simulink model "l512_devel_pps_2016f"  (R2012b)
settings: Solver=ode45  StartTime=0.0  StopTime=15000  RelTol=1e-3
undefined symbols (not defined in the file): sfp
libraries: xbsIndex_r4 x7383, casper_library_misc x259, casper_library_delays x118, xps_library x12, simulink x1
(part 5 of 82)

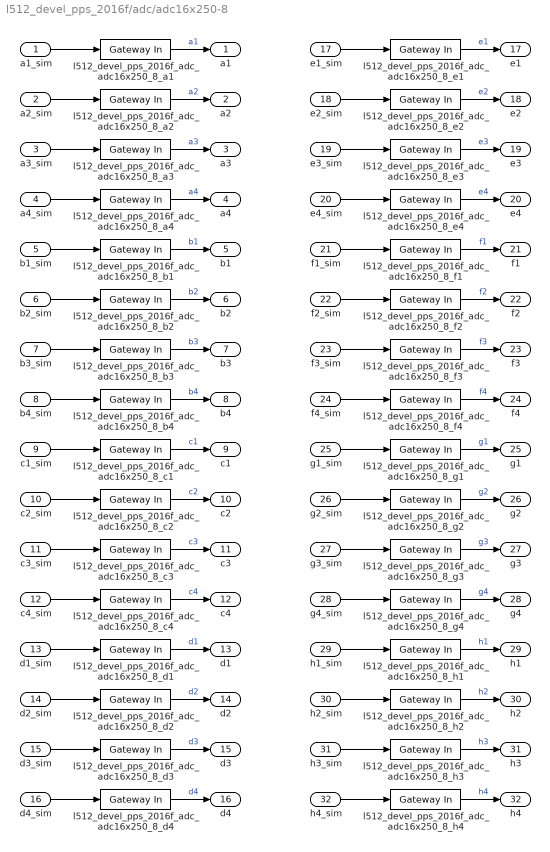
== system l512_devel_pps_2016f/adc/adc16x250-8 ==
  a1_sim : Inport
  a2_sim : Inport  Port=2
  a3_sim : Inport  Port=3
  a4_sim : Inport  Port=4
  b1_sim : Inport  Port=5
  b2_sim : Inport  Port=6
  b3_sim : Inport  Port=7
  b4_sim : Inport  Port=8
  c1_sim : Inport  Port=9
  c2_sim : Inport  Port=10
  c3_sim : Inport  Port=11
  c4_sim : Inport  Port=12
  d1_sim : Inport  Port=13
  d2_sim : Inport  Port=14
  d3_sim : Inport  Port=15
  d4_sim : Inport  Port=16
  e1_sim : Inport  Port=17
  e2_sim : Inport  Port=18
  e3_sim : Inport  Port=19
  e4_sim : Inport  Port=20
  f1_sim : Inport  Port=21
  f2_sim : Inport  Port=22
  f3_sim : Inport  Port=23
  f4_sim : Inport  Port=24
  g1_sim : Inport  Port=25
  g2_sim : Inport  Port=26
  g3_sim : Inport  Port=27
  g4_sim : Inport  Port=28
  h1_sim : Inport  Port=29
  h2_sim : Inport  Port=30
  h3_sim : Inport  Port=31
  h4_sim : Inport  Port=32
  l512_devel_pps_2016f_adc_adc16x250_8_a{1..4} (4 alike) : xbsIndex_r4/Gateway In  gui_display_data_type=Fixed-point  arith_type="Signed  (2's comp)"  n_bits=8  bin_pt=7  preci_type=Single  exp_width=8  frac_width=24  quantization="Round  (unbiased: +/- Inf)"  overflow=Saturate  period=1  dbl_ovrd=off  timing_constraint=None  locs_specified=off  LOCs={}  UseAsADC=off  ADCChannel='1'  inherit_from_input=off  hdl_port=on  block_type=gatewayin
  l512_devel_pps_2016f_adc_adc16x250_8_b{1..4} (4 alike) : xbsIndex_r4/Gateway In  gui_display_data_type=Fixed-point  arith_type="Signed  (2's comp)"  n_bits=8  bin_pt=7  preci_type=Single  exp_width=8  frac_width=24  quantization="Round  (unbiased: +/- Inf)"  overflow=Saturate  period=1  dbl_ovrd=off  timing_constraint=None  locs_specified=off  LOCs={}  UseAsADC=off  ADCChannel='1'  inherit_from_input=off  hdl_port=on  block_type=gatewayin
  l512_devel_pps_2016f_adc_adc16x250_8_c{1..4} (4 alike) : xbsIndex_r4/Gateway In  gui_display_data_type=Fixed-point  arith_type="Signed  (2's comp)"  n_bits=8  bin_pt=7  preci_type=Single  exp_width=8  frac_width=24  quantization="Round  (unbiased: +/- Inf)"  overflow=Saturate  period=1  dbl_ovrd=off  timing_constraint=None  locs_specified=off  LOCs={}  UseAsADC=off  ADCChannel='1'  inherit_from_input=off  hdl_port=on  block_type=gatewayin
  l512_devel_pps_2016f_adc_adc16x250_8_d{1..4} (4 alike) : xbsIndex_r4/Gateway In  gui_display_data_type=Fixed-point  arith_type="Signed  (2's comp)"  n_bits=8  bin_pt=7  preci_type=Single  exp_width=8  frac_width=24  quantization="Round  (unbiased: +/- Inf)"  overflow=Saturate  period=1  dbl_ovrd=off  timing_constraint=None  locs_specified=off  LOCs={}  UseAsADC=off  ADCChannel='1'  inherit_from_input=off  hdl_port=on  block_type=gatewayin
  l512_devel_pps_2016f_adc_adc16x250_8_e{1..4} (4 alike) : xbsIndex_r4/Gateway In  gui_display_data_type=Fixed-point  arith_type="Signed  (2's comp)"  n_bits=8  bin_pt=7  preci_type=Single  exp_width=8  frac_width=24  quantization="Round  (unbiased: +/- Inf)"  overflow=Saturate  period=1  dbl_ovrd=off  timing_constraint=None  locs_specified=off  LOCs={}  UseAsADC=off  ADCChannel='1'  inherit_from_input=off  hdl_port=on  block_type=gatewayin
  l512_devel_pps_2016f_adc_adc16x250_8_f{1..4} (4 alike) : xbsIndex_r4/Gateway In  gui_display_data_type=Fixed-point  arith_type="Signed  (2's comp)"  n_bits=8  bin_pt=7  preci_type=Single  exp_width=8  frac_width=24  quantization="Round  (unbiased: +/- Inf)"  overflow=Saturate  period=1  dbl_ovrd=off  timing_constraint=None  locs_specified=off  LOCs={}  UseAsADC=off  ADCChannel='1'  inherit_from_input=off  hdl_port=on  block_type=gatewayin
  l512_devel_pps_2016f_adc_adc16x250_8_g{1..4} (4 alike) : xbsIndex_r4/Gateway In  gui_display_data_type=Fixed-point  arith_type="Signed  (2's comp)"  n_bits=8  bin_pt=7  preci_type=Single  exp_width=8  frac_width=24  quantization="Round  (unbiased: +/- Inf)"  overflow=Saturate  period=1  dbl_ovrd=off  timing_constraint=None  locs_specified=off  LOCs={}  UseAsADC=off  ADCChannel='1'  inherit_from_input=off  hdl_port=on  block_type=gatewayin
  l512_devel_pps_2016f_adc_adc16x250_8_h{1..4} (4 alike) : xbsIndex_r4/Gateway In  gui_display_data_type=Fixed-point  arith_type="Signed  (2's comp)"  n_bits=8  bin_pt=7  preci_type=Single  exp_width=8  frac_width=24  quantization="Round  (unbiased: +/- Inf)"  overflow=Saturate  period=1  dbl_ovrd=off  timing_constraint=None  locs_specified=off  LOCs={}  UseAsADC=off  ADCChannel='1'  inherit_from_input=off  hdl_port=on  block_type=gatewayin
  a1 : Outport
  a2 : Outport  Port=2
  a3 : Outport  Port=3
  a4 : Outport  Port=4
  b1 : Outport  Port=5
  b2 : Outport  Port=6
  b3 : Outport  Port=7
  b4 : Outport  Port=8
  c1 : Outport  Port=9
  c2 : Outport  Port=10
  c3 : Outport  Port=11
  c4 : Outport  Port=12
  d1 : Outport  Port=13
  d2 : Outport  Port=14
  d3 : Outport  Port=15
  d4 : Outport  Port=16
  e1 : Outport  Port=17
  e2 : Outport  Port=18
  e3 : Outport  Port=19
  e4 : Outport  Port=20
  f1 : Outport  Port=21
  f2 : Outport  Port=22
  f3 : Outport  Port=23
  f4 : Outport  Port=24
  g1 : Outport  Port=25
  g2 : Outport  Port=26
  g3 : Outport  Port=27
  g4 : Outport  Port=28
  h1 : Outport  Port=29
  h2 : Outport  Port=30
  h3 : Outport  Port=31
  h4 : Outport  Port=32
  wires:
  a1_sim/1 -> l512_devel_pps_2016f_adc_adc16x250_8_a1/1
  l512_devel_pps_2016f_adc_adc16x250_8_a1/1 -> a1/1  "a1"
  a2_sim/1 -> l512_devel_pps_2016f_adc_adc16x250_8_a2/1
  l512_devel_pps_2016f_adc_adc16x250_8_a2/1 -> a2/1  "a2"
  a3_sim/1 -> l512_devel_pps_2016f_adc_adc16x250_8_a3/1
  l512_devel_pps_2016f_adc_adc16x250_8_a3/1 -> a3/1  "a3"
  a4_sim/1 -> l512_devel_pps_2016f_adc_adc16x250_8_a4/1
  l512_devel_pps_2016f_adc_adc16x250_8_a4/1 -> a4/1  "a4"
  b1_sim/1 -> l512_devel_pps_2016f_adc_adc16x250_8_b1/1
  l512_devel_pps_2016f_adc_adc16x250_8_b1/1 -> b1/1  "b1"
  b2_sim/1 -> l512_devel_pps_2016f_adc_adc16x250_8_b2/1
  l512_devel_pps_2016f_adc_adc16x250_8_b2/1 -> b2/1  "b2"
  b3_sim/1 -> l512_devel_pps_2016f_adc_adc16x250_8_b3/1
  l512_devel_pps_2016f_adc_adc16x250_8_b3/1 -> b3/1  "b3"
  b4_sim/1 -> l512_devel_pps_2016f_adc_adc16x250_8_b4/1
  l512_devel_pps_2016f_adc_adc16x250_8_b4/1 -> b4/1  "b4"
  c1_sim/1 -> l512_devel_pps_2016f_adc_adc16x250_8_c1/1
  l512_devel_pps_2016f_adc_adc16x250_8_c1/1 -> c1/1  "c1"
  c2_sim/1 -> l512_devel_pps_2016f_adc_adc16x250_8_c2/1
  l512_devel_pps_2016f_adc_adc16x250_8_c2/1 -> c2/1  "c2"
  c3_sim/1 -> l512_devel_pps_2016f_adc_adc16x250_8_c3/1
  l512_devel_pps_2016f_adc_adc16x250_8_c3/1 -> c3/1  "c3"
  c4_sim/1 -> l512_devel_pps_2016f_adc_adc16x250_8_c4/1
  l512_devel_pps_2016f_adc_adc16x250_8_c4/1 -> c4/1  "c4"
  d1_sim/1 -> l512_devel_pps_2016f_adc_adc16x250_8_d1/1
  l512_devel_pps_2016f_adc_adc16x250_8_d1/1 -> d1/1  "d1"
  d2_sim/1 -> l512_devel_pps_2016f_adc_adc16x250_8_d2/1
  l512_devel_pps_2016f_adc_adc16x250_8_d2/1 -> d2/1  "d2"
  d3_sim/1 -> l512_devel_pps_2016f_adc_adc16x250_8_d3/1
  l512_devel_pps_2016f_adc_adc16x250_8_d3/1 -> d3/1  "d3"
  d4_sim/1 -> l512_devel_pps_2016f_adc_adc16x250_8_d4/1
  l512_devel_pps_2016f_adc_adc16x250_8_d4/1 -> d4/1  "d4"
  e1_sim/1 -> l512_devel_pps_2016f_adc_adc16x250_8_e1/1
  l512_devel_pps_2016f_adc_adc16x250_8_e1/1 -> e1/1  "e1"
  e2_sim/1 -> l512_devel_pps_2016f_adc_adc16x250_8_e2/1
  l512_devel_pps_2016f_adc_adc16x250_8_e2/1 -> e2/1  "e2"
  e3_sim/1 -> l512_devel_pps_2016f_adc_adc16x250_8_e3/1
  l512_devel_pps_2016f_adc_adc16x250_8_e3/1 -> e3/1  "e3"
  e4_sim/1 -> l512_devel_pps_2016f_adc_adc16x250_8_e4/1
  l512_devel_pps_2016f_adc_adc16x250_8_e4/1 -> e4/1  "e4"
  f1_sim/1 -> l512_devel_pps_2016f_adc_adc16x250_8_f1/1
  l512_devel_pps_2016f_adc_adc16x250_8_f1/1 -> f1/1  "f1"
  f2_sim/1 -> l512_devel_pps_2016f_adc_adc16x250_8_f2/1
  l512_devel_pps_2016f_adc_adc16x250_8_f2/1 -> f2/1  "f2"
  f3_sim/1 -> l512_devel_pps_2016f_adc_adc16x250_8_f3/1
  l512_devel_pps_2016f_adc_adc16x250_8_f3/1 -> f3/1  "f3"
  f4_sim/1 -> l512_devel_pps_2016f_adc_adc16x250_8_f4/1
  l512_devel_pps_2016f_adc_adc16x250_8_f4/1 -> f4/1  "f4"
  g1_sim/1 -> l512_devel_pps_2016f_adc_adc16x250_8_g1/1
  l512_devel_pps_2016f_adc_adc16x250_8_g1/1 -> g1/1  "g1"
  g2_sim/1 -> l512_devel_pps_2016f_adc_adc16x250_8_g2/1
  l512_devel_pps_2016f_adc_adc16x250_8_g2/1 -> g2/1  "g2"
  g3_sim/1 -> l512_devel_pps_2016f_adc_adc16x250_8_g3/1
  l512_devel_pps_2016f_adc_adc16x250_8_g3/1 -> g3/1  "g3"
  g4_sim/1 -> l512_devel_pps_2016f_adc_adc16x250_8_g4/1
  l512_devel_pps_2016f_adc_adc16x250_8_g4/1 -> g4/1  "g4"
  h1_sim/1 -> l512_devel_pps_2016f_adc_adc16x250_8_h1/1
  l512_devel_pps_2016f_adc_adc16x250_8_h1/1 -> h1/1  "h1"
  h2_sim/1 -> l512_devel_pps_2016f_adc_adc16x250_8_h2/1
  l512_devel_pps_2016f_adc_adc16x250_8_h2/1 -> h2/1  "h2"
  h3_sim/1 -> l512_devel_pps_2016f_adc_adc16x250_8_h3/1
  l512_devel_pps_2016f_adc_adc16x250_8_h3/1 -> h3/1  "h3"
  h4_sim/1 -> l512_devel_pps_2016f_adc_adc16x250_8_h4/1
  l512_devel_pps_2016f_adc_adc16x250_8_h4/1 -> h4/1  "h4"

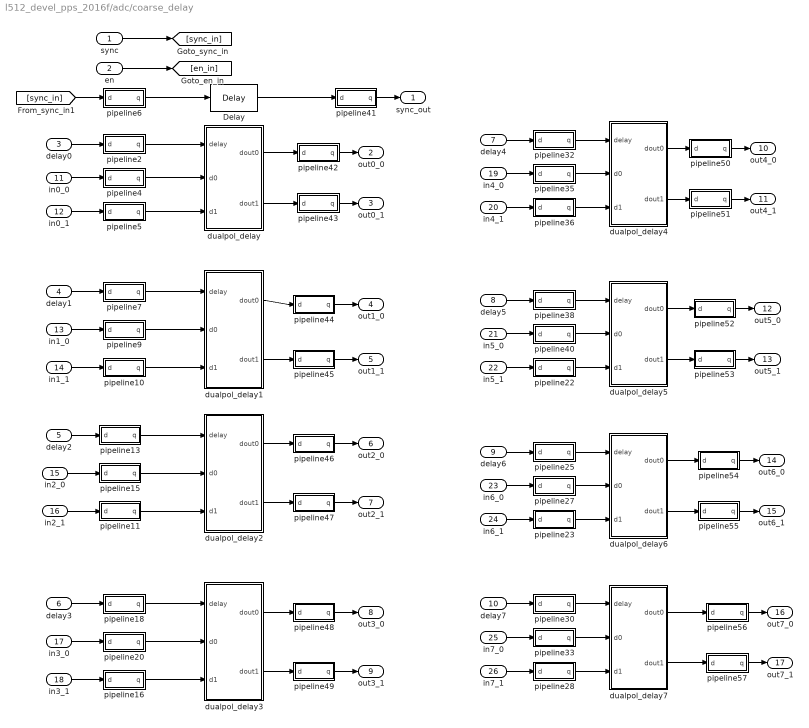
== system l512_devel_pps_2016f/adc/coarse_delay ==
  sync : Inport
  en : Inport  Port=2
  delay0 : Inport  Port=3
  delay1 : Inport  Port=4
  delay2 : Inport  Port=5
  delay3 : Inport  Port=6
  delay4 : Inport  Port=7
  delay5 : Inport  Port=8
  delay6 : Inport  Port=9
  delay7 : Inport  Port=10
  in0_0 : Inport  Port=11
  in0_1 : Inport  Port=12
  in1_0 : Inport  Port=13
  in1_1 : Inport  Port=14
  in2_0 : Inport  Port=15
  in2_1 : Inport  Port=16
  in3_0 : Inport  Port=17
  in3_1 : Inport  Port=18
  in4_0 : Inport  Port=19
  in4_1 : Inport  Port=20
  in5_0 : Inport  Port=21
  in5_1 : Inport  Port=22
  in6_0 : Inport  Port=23
  in6_1 : Inport  Port=24
  in7_0 : Inport  Port=25
  in7_1 : Inport  Port=26
  Delay : xbsIndex_r4/Delay  rst=off  infoeditControl=Selection of Reset will increase slice count due to use of real FFs and instead of SRLs  en=off  latency=3  dbl_ovrd=off  reg_retiming=off  block_type=delay
  dualpol_delay : Subsystem
  dualpol_delay1 : Subsystem
  dualpol_delay2 : Subsystem
  dualpol_delay3 : Subsystem
  dualpol_delay4 : Subsystem
  dualpol_delay5 : Subsystem
  dualpol_delay6 : Subsystem
  dualpol_delay7 : Subsystem
  pipeline10 : Subsystem  AncestorBlock=casper_library_delays/pipeline  mask(pipeline){latency=1}
      mask help:
      | An explicitly laid-out delay line to avoid mapping to SRL16s
      | for use in pipelining to help achieve timing closure.
      mask init:
      | pipeline_init(gcb,'latency',latency);
      settings: AttributesFormatString=Latency = %<latency>
      mask Display:
      | port_label('input', 1, 'd');
      | port_label('output', 1, 'q');
      | disp(['Z^-', num2str(latency)]);
  pipeline11 : Subsystem  AncestorBlock=casper_library_delays/pipeline  mask(pipeline){latency=1}
      mask help:
      | An explicitly laid-out delay line to avoid mapping to SRL16s
      | for use in pipelining to help achieve timing closure.
      mask init:
      | pipeline_init(gcb,'latency',latency);
      settings: AttributesFormatString=Latency = %<latency>
      mask Display:
      | port_label('input', 1, 'd');
      | port_label('output', 1, 'q');
      | disp(['Z^-', num2str(latency)]);
  pipeline13 : Subsystem  AncestorBlock=casper_library_delays/pipeline  mask(pipeline){latency=1}
      mask help:
      | An explicitly laid-out delay line to avoid mapping to SRL16s
      | for use in pipelining to help achieve timing closure.
      mask init:
      | pipeline_init(gcb,'latency',latency);
      settings: AttributesFormatString=Latency = %<latency>
      mask Display:
      | port_label('input', 1, 'd');
      | port_label('output', 1, 'q');
      | disp(['Z^-', num2str(latency)]);
  pipeline15 : Subsystem  AncestorBlock=casper_library_delays/pipeline  mask(pipeline){latency=1}
      mask help:
      | An explicitly laid-out delay line to avoid mapping to SRL16s
      | for use in pipelining to help achieve timing closure.
      mask init:
      | pipeline_init(gcb,'latency',latency);
      settings: AttributesFormatString=Latency = %<latency>
      mask Display:
      | port_label('input', 1, 'd');
      | port_label('output', 1, 'q');
      | disp(['Z^-', num2str(latency)]);
  pipeline16 : Subsystem  AncestorBlock=casper_library_delays/pipeline  mask(pipeline){latency=1}
      mask help:
      | An explicitly laid-out delay line to avoid mapping to SRL16s
      | for use in pipelining to help achieve timing closure.
      mask init:
      | pipeline_init(gcb,'latency',latency);
      settings: AttributesFormatString=Latency = %<latency>
      mask Display:
      | port_label('input', 1, 'd');
      | port_label('output', 1, 'q');
      | disp(['Z^-', num2str(latency)]);
  pipeline18 : Subsystem  AncestorBlock=casper_library_delays/pipeline  mask(pipeline){latency=1}
      mask help:
      | An explicitly laid-out delay line to avoid mapping to SRL16s
      | for use in pipelining to help achieve timing closure.
      mask init:
      | pipeline_init(gcb,'latency',latency);
      settings: AttributesFormatString=Latency = %<latency>
      mask Display:
      | port_label('input', 1, 'd');
      | port_label('output', 1, 'q');
      | disp(['Z^-', num2str(latency)]);
  pipeline2 : Subsystem  AncestorBlock=casper_library_delays/pipeline  mask(pipeline){latency=1}
      mask help:
      | An explicitly laid-out delay line to avoid mapping to SRL16s
      | for use in pipelining to help achieve timing closure.
      mask init:
      | pipeline_init(gcb,'latency',latency);
      settings: AttributesFormatString=Latency = %<latency>
      mask Display:
      | port_label('input', 1, 'd');
      | port_label('output', 1, 'q');
      | disp(['Z^-', num2str(latency)]);
  pipeline20 : Subsystem  AncestorBlock=casper_library_delays/pipeline  mask(pipeline){latency=1}
      mask help:
      | An explicitly laid-out delay line to avoid mapping to SRL16s
      | for use in pipelining to help achieve timing closure.
      mask init:
      | pipeline_init(gcb,'latency',latency);
      settings: AttributesFormatString=Latency = %<latency>
      mask Display:
      | port_label('input', 1, 'd');
      | port_label('output', 1, 'q');
      | disp(['Z^-', num2str(latency)]);
  pipeline22 : Subsystem  AncestorBlock=casper_library_delays/pipeline  mask(pipeline){latency=1}
      mask help:
      | An explicitly laid-out delay line to avoid mapping to SRL16s
      | for use in pipelining to help achieve timing closure.
      mask init:
      | pipeline_init(gcb,'latency',latency);
      settings: AttributesFormatString=Latency = %<latency>
      mask Display:
      | port_label('input', 1, 'd');
      | port_label('output', 1, 'q');
      | disp(['Z^-', num2str(latency)]);
  pipeline23 : Subsystem  AncestorBlock=casper_library_delays/pipeline  mask(pipeline){latency=1}
      mask help:
      | An explicitly laid-out delay line to avoid mapping to SRL16s
      | for use in pipelining to help achieve timing closure.
      mask init:
      | pipeline_init(gcb,'latency',latency);
      settings: AttributesFormatString=Latency = %<latency>
      mask Display:
      | port_label('input', 1, 'd');
      | port_label('output', 1, 'q');
      | disp(['Z^-', num2str(latency)]);
  pipeline25 : Subsystem  AncestorBlock=casper_library_delays/pipeline  mask(pipeline){latency=1}
      mask help:
      | An explicitly laid-out delay line to avoid mapping to SRL16s
      | for use in pipelining to help achieve timing closure.
      mask init:
      | pipeline_init(gcb,'latency',latency);
      settings: AttributesFormatString=Latency = %<latency>
      mask Display:
      | port_label('input', 1, 'd');
      | port_label('output', 1, 'q');
      | disp(['Z^-', num2str(latency)]);
  pipeline27 : Subsystem  AncestorBlock=casper_library_delays/pipeline  mask(pipeline){latency=1}
      mask help:
      | An explicitly laid-out delay line to avoid mapping to SRL16s
      | for use in pipelining to help achieve timing closure.
      mask init:
      | pipeline_init(gcb,'latency',latency);
      settings: AttributesFormatString=Latency = %<latency>
      mask Display:
      | port_label('input', 1, 'd');
      | port_label('output', 1, 'q');
      | disp(['Z^-', num2str(latency)]);
  pipeline28 : Subsystem  AncestorBlock=casper_library_delays/pipeline  mask(pipeline){latency=1}
      mask help:
      | An explicitly laid-out delay line to avoid mapping to SRL16s
      | for use in pipelining to help achieve timing closure.
      mask init:
      | pipeline_init(gcb,'latency',latency);
      settings: AttributesFormatString=Latency = %<latency>
      mask Display:
      | port_label('input', 1, 'd');
      | port_label('output', 1, 'q');
      | disp(['Z^-', num2str(latency)]);
  pipeline30 : Subsystem  AncestorBlock=casper_library_delays/pipeline  mask(pipeline){latency=1}
      mask help:
      | An explicitly laid-out delay line to avoid mapping to SRL16s
      | for use in pipelining to help achieve timing closure.
      mask init:
      | pipeline_init(gcb,'latency',latency);
      settings: AttributesFormatString=Latency = %<latency>
      mask Display:
      | port_label('input', 1, 'd');
      | port_label('output', 1, 'q');
      | disp(['Z^-', num2str(latency)]);
  pipeline32 : Subsystem  AncestorBlock=casper_library_delays/pipeline  mask(pipeline){latency=1}
      mask help:
      | An explicitly laid-out delay line to avoid mapping to SRL16s
      | for use in pipelining to help achieve timing closure.
      mask init:
      | pipeline_init(gcb,'latency',latency);
      settings: AttributesFormatString=Latency = %<latency>
      mask Display:
      | port_label('input', 1, 'd');
      | port_label('output', 1, 'q');
      | disp(['Z^-', num2str(latency)]);
  pipeline33 : Subsystem  AncestorBlock=casper_library_delays/pipeline  mask(pipeline){latency=1}
      mask help:
      | An explicitly laid-out delay line to avoid mapping to SRL16s
      | for use in pipelining to help achieve timing closure.
      mask init:
      | pipeline_init(gcb,'latency',latency);
      settings: AttributesFormatString=Latency = %<latency>
      mask Display:
      | port_label('input', 1, 'd');
      | port_label('output', 1, 'q');
      | disp(['Z^-', num2str(latency)]);
  pipeline35 : Subsystem  AncestorBlock=casper_library_delays/pipeline  mask(pipeline){latency=1}
      mask help:
      | An explicitly laid-out delay line to avoid mapping to SRL16s
      | for use in pipelining to help achieve timing closure.
      mask init:
      | pipeline_init(gcb,'latency',latency);
      settings: AttributesFormatString=Latency = %<latency>
      mask Display:
      | port_label('input', 1, 'd');
      | port_label('output', 1, 'q');
      | disp(['Z^-', num2str(latency)]);
  pipeline36 : Subsystem  AncestorBlock=casper_library_delays/pipeline  mask(pipeline){latency=1}
      mask help:
      | An explicitly laid-out delay line to avoid mapping to SRL16s
      | for use in pipelining to help achieve timing closure.
      mask init:
      | pipeline_init(gcb,'latency',latency);
      settings: AttributesFormatString=Latency = %<latency>
      mask Display:
      | port_label('input', 1, 'd');
      | port_label('output', 1, 'q');
      | disp(['Z^-', num2str(latency)]);
  pipeline38 : Subsystem  AncestorBlock=casper_library_delays/pipeline  mask(pipeline){latency=1}
      mask help:
      | An explicitly laid-out delay line to avoid mapping to SRL16s
      | for use in pipelining to help achieve timing closure.
      mask init:
      | pipeline_init(gcb,'latency',latency);
      settings: AttributesFormatString=Latency = %<latency>
      mask Display:
      | port_label('input', 1, 'd');
      | port_label('output', 1, 'q');
      | disp(['Z^-', num2str(latency)]);
  pipeline4 : Subsystem  AncestorBlock=casper_library_delays/pipeline  mask(pipeline){latency=1}
      mask help:
      | An explicitly laid-out delay line to avoid mapping to SRL16s
      | for use in pipelining to help achieve timing closure.
      mask init:
      | pipeline_init(gcb,'latency',latency);
      settings: AttributesFormatString=Latency = %<latency>
      mask Display:
      | port_label('input', 1, 'd');
      | port_label('output', 1, 'q');
      | disp(['Z^-', num2str(latency)]);
  pipeline40 : Subsystem  AncestorBlock=casper_library_delays/pipeline  mask(pipeline){latency=1}
      mask help:
      | An explicitly laid-out delay line to avoid mapping to SRL16s
      | for use in pipelining to help achieve timing closure.
      mask init:
      | pipeline_init(gcb,'latency',latency);
      settings: AttributesFormatString=Latency = %<latency>
      mask Display:
      | port_label('input', 1, 'd');
      | port_label('output', 1, 'q');
      | disp(['Z^-', num2str(latency)]);
  pipeline41 : Subsystem  AncestorBlock=casper_library_delays/pipeline  mask(pipeline){latency=1}
      mask help:
      | An explicitly laid-out delay line to avoid mapping to SRL16s
      | for use in pipelining to help achieve timing closure.
      mask init:
      | pipeline_init(gcb,'latency',latency);
      settings: AttributesFormatString=Latency = %<latency>
      mask Display:
      | port_label('input', 1, 'd');
      | port_label('output', 1, 'q');
      | disp(['Z^-', num2str(latency)]);
  pipeline42 : Subsystem  AncestorBlock=casper_library_delays/pipeline  mask(pipeline){latency=1}
      mask help:
      | An explicitly laid-out delay line to avoid mapping to SRL16s
      | for use in pipelining to help achieve timing closure.
      mask init:
      | pipeline_init(gcb,'latency',latency);
      settings: AttributesFormatString=Latency = %<latency>
      mask Display:
      | port_label('input', 1, 'd');
      | port_label('output', 1, 'q');
      | disp(['Z^-', num2str(latency)]);
  pipeline43 : Subsystem  AncestorBlock=casper_library_delays/pipeline  mask(pipeline){latency=1}
      mask help:
      | An explicitly laid-out delay line to avoid mapping to SRL16s
      | for use in pipelining to help achieve timing closure.
      mask init:
      | pipeline_init(gcb,'latency',latency);
      settings: AttributesFormatString=Latency = %<latency>
      mask Display:
      | port_label('input', 1, 'd');
      | port_label('output', 1, 'q');
      | disp(['Z^-', num2str(latency)]);
  pipeline44 : Subsystem  AncestorBlock=casper_library_delays/pipeline  mask(pipeline){latency=1}
      mask help:
      | An explicitly laid-out delay line to avoid mapping to SRL16s
      | for use in pipelining to help achieve timing closure.
      mask init:
      | pipeline_init(gcb,'latency',latency);
      settings: AttributesFormatString=Latency = %<latency>
      mask Display:
      | port_label('input', 1, 'd');
      | port_label('output', 1, 'q');
      | disp(['Z^-', num2str(latency)]);
  pipeline45 : Subsystem  AncestorBlock=casper_library_delays/pipeline  mask(pipeline){latency=1}
      mask help:
      | An explicitly laid-out delay line to avoid mapping to SRL16s
      | for use in pipelining to help achieve timing closure.
      mask init:
      | pipeline_init(gcb,'latency',latency);
      settings: AttributesFormatString=Latency = %<latency>
      mask Display:
      | port_label('input', 1, 'd');
      | port_label('output', 1, 'q');
      | disp(['Z^-', num2str(latency)]);
  pipeline46 : Subsystem  AncestorBlock=casper_library_delays/pipeline  mask(pipeline){latency=1}
      mask help:
      | An explicitly laid-out delay line to avoid mapping to SRL16s
      | for use in pipelining to help achieve timing closure.
      mask init:
      | pipeline_init(gcb,'latency',latency);
      settings: AttributesFormatString=Latency = %<latency>
      mask Display:
      | port_label('input', 1, 'd');
      | port_label('output', 1, 'q');
      | disp(['Z^-', num2str(latency)]);
  pipeline47 : Subsystem  AncestorBlock=casper_library_delays/pipeline  mask(pipeline){latency=1}
      mask help:
      | An explicitly laid-out delay line to avoid mapping to SRL16s
      | for use in pipelining to help achieve timing closure.
      mask init:
      | pipeline_init(gcb,'latency',latency);
      settings: AttributesFormatString=Latency = %<latency>
      mask Display:
      | port_label('input', 1, 'd');
      | port_label('output', 1, 'q');
      | disp(['Z^-', num2str(latency)]);
  pipeline48 : Subsystem  AncestorBlock=casper_library_delays/pipeline  mask(pipeline){latency=1}
      mask help:
      | An explicitly laid-out delay line to avoid mapping to SRL16s
      | for use in pipelining to help achieve timing closure.
      mask init:
      | pipeline_init(gcb,'latency',latency);
      settings: AttributesFormatString=Latency = %<latency>
      mask Display:
      | port_label('input', 1, 'd');
      | port_label('output', 1, 'q');
      | disp(['Z^-', num2str(latency)]);
  pipeline49 : Subsystem  AncestorBlock=casper_library_delays/pipeline  mask(pipeline){latency=1}
      mask help:
      | An explicitly laid-out delay line to avoid mapping to SRL16s
      | for use in pipelining to help achieve timing closure.
      mask init:
      | pipeline_init(gcb,'latency',latency);
      settings: AttributesFormatString=Latency = %<latency>
      mask Display:
      | port_label('input', 1, 'd');
      | port_label('output', 1, 'q');
      | disp(['Z^-', num2str(latency)]);
  pipeline5 : Subsystem  AncestorBlock=casper_library_delays/pipeline  mask(pipeline){latency=1}
      mask help:
      | An explicitly laid-out delay line to avoid mapping to SRL16s
      | for use in pipelining to help achieve timing closure.
      mask init:
      | pipeline_init(gcb,'latency',latency);
      settings: AttributesFormatString=Latency = %<latency>
      mask Display:
      | port_label('input', 1, 'd');
      | port_label('output', 1, 'q');
      | disp(['Z^-', num2str(latency)]);
  pipeline50 : Subsystem  AncestorBlock=casper_library_delays/pipeline  mask(pipeline){latency=1}
      mask help:
      | An explicitly laid-out delay line to avoid mapping to SRL16s
      | for use in pipelining to help achieve timing closure.
      mask init:
      | pipeline_init(gcb,'latency',latency);
      settings: AttributesFormatString=Latency = %<latency>
      mask Display:
      | port_label('input', 1, 'd');
      | port_label('output', 1, 'q');
      | disp(['Z^-', num2str(latency)]);
  pipeline51 : Subsystem  AncestorBlock=casper_library_delays/pipeline  mask(pipeline){latency=1}
      mask help:
      | An explicitly laid-out delay line to avoid mapping to SRL16s
      | for use in pipelining to help achieve timing closure.
      mask init:
      | pipeline_init(gcb,'latency',latency);
      settings: AttributesFormatString=Latency = %<latency>
      mask Display:
      | port_label('input', 1, 'd');
      | port_label('output', 1, 'q');
      | disp(['Z^-', num2str(latency)]);
  pipeline52 : Subsystem  AncestorBlock=casper_library_delays/pipeline  mask(pipeline){latency=1}
      mask help:
      | An explicitly laid-out delay line to avoid mapping to SRL16s
      | for use in pipelining to help achieve timing closure.
      mask init:
      | pipeline_init(gcb,'latency',latency);
      settings: AttributesFormatString=Latency = %<latency>
      mask Display:
      | port_label('input', 1, 'd');
      | port_label('output', 1, 'q');
      | disp(['Z^-', num2str(latency)]);
  pipeline53 : Subsystem  AncestorBlock=casper_library_delays/pipeline  mask(pipeline){latency=1}
      mask help:
      | An explicitly laid-out delay line to avoid mapping to SRL16s
      | for use in pipelining to help achieve timing closure.
      mask init:
      | pipeline_init(gcb,'latency',latency);
      settings: AttributesFormatString=Latency = %<latency>
      mask Display:
      | port_label('input', 1, 'd');
      | port_label('output', 1, 'q');
      | disp(['Z^-', num2str(latency)]);
  pipeline54 : Subsystem  AncestorBlock=casper_library_delays/pipeline  mask(pipeline){latency=1}
      mask help:
      | An explicitly laid-out delay line to avoid mapping to SRL16s
      | for use in pipelining to help achieve timing closure.
      mask init:
      | pipeline_init(gcb,'latency',latency);
      settings: AttributesFormatString=Latency = %<latency>
      mask Display:
      | port_label('input', 1, 'd');
      | port_label('output', 1, 'q');
      | disp(['Z^-', num2str(latency)]);
  pipeline55 : Subsystem  AncestorBlock=casper_library_delays/pipeline  mask(pipeline){latency=1}
      mask help:
      | An explicitly laid-out delay line to avoid mapping to SRL16s
      | for use in pipelining to help achieve timing closure.
      mask init:
      | pipeline_init(gcb,'latency',latency);
      settings: AttributesFormatString=Latency = %<latency>
      mask Display:
      | port_label('input', 1, 'd');
      | port_label('output', 1, 'q');
      | disp(['Z^-', num2str(latency)]);
  pipeline56 : Subsystem  AncestorBlock=casper_library_delays/pipeline  mask(pipeline){latency=1}
      mask help:
      | An explicitly laid-out delay line to avoid mapping to SRL16s
      | for use in pipelining to help achieve timing closure.
      mask init:
      | pipeline_init(gcb,'latency',latency);
      settings: AttributesFormatString=Latency = %<latency>
      mask Display:
      | port_label('input', 1, 'd');
      | port_label('output', 1, 'q');
      | disp(['Z^-', num2str(latency)]);
  pipeline57 : Subsystem  AncestorBlock=casper_library_delays/pipeline  mask(pipeline){latency=1}
      mask help:
      | An explicitly laid-out delay line to avoid mapping to SRL16s
      | for use in pipelining to help achieve timing closure.
      mask init:
      | pipeline_init(gcb,'latency',latency);
      settings: AttributesFormatString=Latency = %<latency>
      mask Display:
      | port_label('input', 1, 'd');
      | port_label('output', 1, 'q');
      | disp(['Z^-', num2str(latency)]);
  pipeline6 : Subsystem  AncestorBlock=casper_library_delays/pipeline  mask(pipeline){latency=1}
      mask help:
      | An explicitly laid-out delay line to avoid mapping to SRL16s
      | for use in pipelining to help achieve timing closure.
      mask init:
      | pipeline_init(gcb,'latency',latency);
      settings: AttributesFormatString=Latency = %<latency>
      mask Display:
      | port_label('input', 1, 'd');
      | port_label('output', 1, 'q');
      | disp(['Z^-', num2str(latency)]);
  pipeline7 : Subsystem  AncestorBlock=casper_library_delays/pipeline  mask(pipeline){latency=1}
      mask help:
      | An explicitly laid-out delay line to avoid mapping to SRL16s
      | for use in pipelining to help achieve timing closure.
      mask init:
      | pipeline_init(gcb,'latency',latency);
      settings: AttributesFormatString=Latency = %<latency>
      mask Display:
      | port_label('input', 1, 'd');
      | port_label('output', 1, 'q');
      | disp(['Z^-', num2str(latency)]);
  pipeline9 : Subsystem  AncestorBlock=casper_library_delays/pipeline  mask(pipeline){latency=1}
      mask help:
      | An explicitly laid-out delay line to avoid mapping to SRL16s
      | for use in pipelining to help achieve timing closure.
      mask init:
      | pipeline_init(gcb,'latency',latency);
      settings: AttributesFormatString=Latency = %<latency>
      mask Display:
      | port_label('input', 1, 'd');
      | port_label('output', 1, 'q');
      | disp(['Z^-', num2str(latency)]);
  sync_out : Outport
  out0_0 : Outport  Port=2
  out0_1 : Outport  Port=3
  out1_0 : Outport  Port=4
  out1_1 : Outport  Port=5
  out2_0 : Outport  Port=6
  out2_1 : Outport  Port=7
  out3_0 : Outport  Port=8
  out3_1 : Outport  Port=9
  out4_0 : Outport  Port=10
  out4_1 : Outport  Port=11
  out5_0 : Outport  Port=12
  out5_1 : Outport  Port=13
  out6_0 : Outport  Port=14
  out6_1 : Outport  Port=15
  out7_0 : Outport  Port=16
  out7_1 : Outport  Port=17
  wires:
  dualpol_delay/1(dout0) -> pipeline42/1(d)
  dualpol_delay/2(dout1) -> pipeline43/1(d)
  pipeline6/1(q) -> Delay/1
  sync/1 -> [sync_in]
  en/1 -> [en_in]
  in0_0/1 -> pipeline4/1(d)
  delay0/1 -> pipeline2/1(d)
  in0_1/1 -> pipeline5/1(d)
  dualpol_delay1/1(dout0) -> pipeline44/1(d)
  dualpol_delay1/2(dout1) -> pipeline45/1(d)
  [sync_in] -> pipeline6/1(d)
  in1_0/1 -> pipeline9/1(d)
  delay1/1 -> pipeline7/1(d)
  in1_1/1 -> pipeline10/1(d)
  dualpol_delay2/1(dout0) -> pipeline46/1(d)
  dualpol_delay2/2(dout1) -> pipeline47/1(d)
  in2_0/1 -> pipeline15/1(d)
  delay2/1 -> pipeline13/1(d)
  in2_1/1 -> pipeline11/1(d)
  dualpol_delay3/1(dout0) -> pipeline48/1(d)
  dualpol_delay3/2(dout1) -> pipeline49/1(d)
  in3_0/1 -> pipeline20/1(d)
  delay3/1 -> pipeline18/1(d)
  in3_1/1 -> pipeline16/1(d)
  dualpol_delay4/1(dout0) -> pipeline50/1(d)
  dualpol_delay4/2(dout1) -> pipeline51/1(d)
  in4_0/1 -> pipeline35/1(d)
  delay4/1 -> pipeline32/1(d)
  in4_1/1 -> pipeline36/1(d)
  dualpol_delay5/1(dout0) -> pipeline52/1(d)
  dualpol_delay5/2(dout1) -> pipeline53/1(d)
  in5_0/1 -> pipeline40/1(d)
  delay5/1 -> pipeline38/1(d)
  in5_1/1 -> pipeline22/1(d)
  dualpol_delay6/1(dout0) -> pipeline54/1(d)
  dualpol_delay6/2(dout1) -> pipeline55/1(d)
  in6_0/1 -> pipeline27/1(d)
  delay6/1 -> pipeline25/1(d)
  in6_1/1 -> pipeline23/1(d)
  dualpol_delay7/1(dout0) -> pipeline56/1(d)
  dualpol_delay7/2(dout1) -> pipeline57/1(d)
  in7_0/1 -> pipeline33/1(d)
  delay7/1 -> pipeline30/1(d)
  in7_1/1 -> pipeline28/1(d)
  pipeline9/1(q) -> dualpol_delay1/2(d0)
  pipeline10/1(q) -> dualpol_delay1/3(d1)
  pipeline7/1(q) -> dualpol_delay1/1(delay)
  pipeline11/1(q) -> dualpol_delay2/3(d1)
  pipeline15/1(q) -> dualpol_delay2/2(d0)
  pipeline13/1(q) -> dualpol_delay2/1(delay)
  pipeline20/1(q) -> dualpol_delay3/2(d0)
  pipeline16/1(q) -> dualpol_delay3/3(d1)
  pipeline18/1(q) -> dualpol_delay3/1(delay)
  pipeline22/1(q) -> dualpol_delay5/3(d1)
  pipeline23/1(q) -> dualpol_delay6/3(d1)
  pipeline25/1(q) -> dualpol_delay6/1(delay)
  pipeline27/1(q) -> dualpol_delay6/2(d0)
  pipeline28/1(q) -> dualpol_delay7/3(d1)
  pipeline32/1(q) -> dualpol_delay4/1(delay)
  pipeline30/1(q) -> dualpol_delay7/1(delay)
  pipeline33/1(q) -> dualpol_delay7/2(d0)
  pipeline35/1(q) -> dualpol_delay4/2(d0)
  pipeline36/1(q) -> dualpol_delay4/3(d1)
  pipeline38/1(q) -> dualpol_delay5/1(delay)
  pipeline40/1(q) -> dualpol_delay5/2(d0)
  pipeline41/1(q) -> sync_out/1
  pipeline42/1(q) -> out0_0/1
  pipeline43/1(q) -> out0_1/1
  pipeline45/1(q) -> out1_1/1
  pipeline44/1(q) -> out1_0/1
  pipeline46/1(q) -> out2_0/1
  pipeline47/1(q) -> out2_1/1
  pipeline48/1(q) -> out3_0/1
  pipeline49/1(q) -> out3_1/1
  pipeline51/1(q) -> out4_1/1
  pipeline50/1(q) -> out4_0/1
  pipeline53/1(q) -> out5_1/1
  pipeline52/1(q) -> out5_0/1
  pipeline55/1(q) -> out6_1/1
  pipeline54/1(q) -> out6_0/1
  pipeline56/1(q) -> out7_0/1
  pipeline57/1(q) -> out7_1/1
  pipeline2/1(q) -> dualpol_delay/1(delay)
  pipeline4/1(q) -> dualpol_delay/2(d0)
  pipeline5/1(q) -> dualpol_delay/3(d1)
  Delay/1 -> pipeline41/1(d)
